simulink model "martins_version_wconv_wdc_wWT"  (R2023b)
settings: Solver=VariableStepAuto  StartTime=0.0  StopTime=30  RelTol=1.0e-3
undefined symbols (not defined in the file): C_dc, c_drt, c_f, C_hv_km, C_p_opt, Cagg, DiscIntNeverNeededParam, G_dc_denom, G_dc_num, H_gen, H_vsm, H_WTR, Ibase_hv, Ibase_lv, Ibase_mv, k_AD, k_d_vsm, k_decouple, k_drt, k_ffv, k_ic, k_idc, k_mod, k_p_p_vsm, k_p_q_vsm, k_pc, k_pdc, K_pitch, ki_dc, KI_LL, ki_q, kp_dc, KP_LL, kslope_VSC, L_comp, L_d, l_f, l_f_si1, l_grid, L_hv_km, L_q, l_t_ehvhv, l_t_hvmv, l_t_mvlv, L_Virt, Lagg, lambda_opt, Lbase1v, length_export, omega_nom, omega_WTR_min, omega_WTR_n, omega_WTR_sl, P_aero_0, phase_shift_test_state, phase_shifts, pie_export, pitch_max, pitch_min, Pitchanglevector ... (+40)
libraries: slpidlib x9, spsFirstOrderFilterLib x3, simulink x1, spsSampleandHoldLib x1, spspowerguiLib x1
(part 2 of 4)

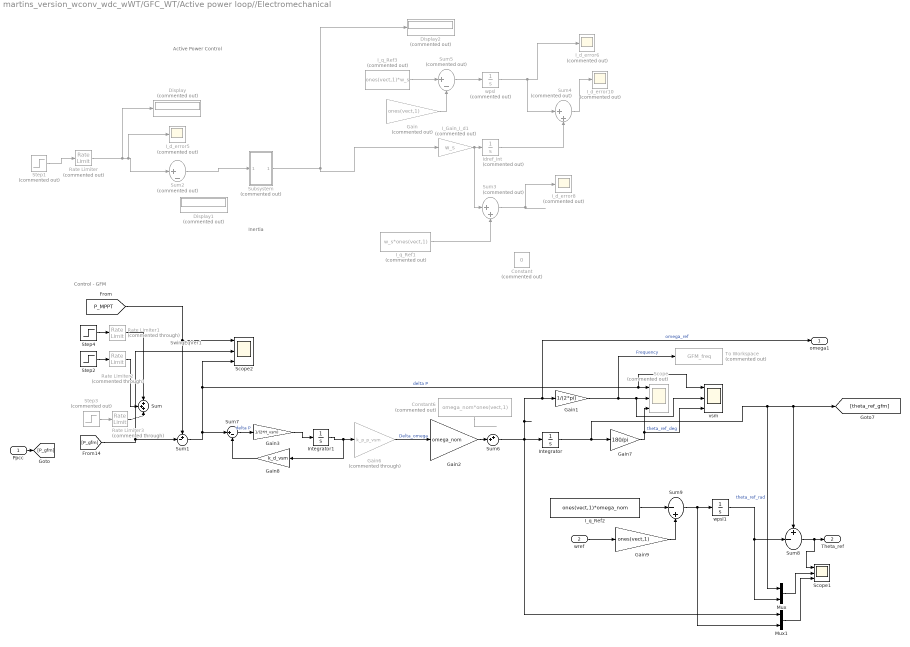
== system martins_version_wconv_wdc_wWT/GFC_WT/Active power loop//Electromechanical ==
  note: SwingEqVer1
  note: Active Power Control
  note: Inertia
  note: Control - GFM
  Ppcc : Inport  PortDimensions=vect
  wref : Inport  Port=2
  Constant : Constant  Commented=on  Value=0
  Constant6 : Constant  Commented=on  Value=omega_nom*ones(vect,1)
  Display : Display  Commented=on
  Display1 : Display  Commented=on
  Display2 : Display  Commented=on
  Gain : Gain  Commented=on  Gain=ones(vect,1)
  Gain1 : Gain  Gain=1/(2*pi)
  Gain2 : Gain  Gain=omega_nom
  Gain3 : Gain  Gain=1/(2*H_vsm)
  Gain6 : Gain  Commented=through  Gain=k_p_p_vsm
  Gain7 : Gain  Gain=180/pi
  Gain8 : Gain  Gain=k_d_vsm
  Gain9 : Gain  Gain=ones(vect,1)
  I_Gain_I_d1 : Gain  Commented=on  Gain=w_s
  I_d_error{5..6,8,10} (4 alike) : Scope  Commented=on
  I_q_Ref1 : Constant  Commented=on  Value=w_s*ones(vect,1)  SampleTime=-1
  I_q_Ref2 : Constant  Value=ones(vect,1)*omega_nom  SampleTime=-1
  I_q_Ref3 : Constant  Commented=on  Value=ones(vect,1)*w_s  SampleTime=-1
  "Idref_int " : Integrator  Commented=on  UpperSaturationLimit=300  LowerSaturationLimit=-100
  Integrator : Integrator  WrappedStateUpperValue=2*pi  WrappedStateLowerValue=0
  Integrator1 : Integrator
  Mux : Mux  Inputs=2
  Mux1 : Mux  Inputs=2
  Rate Limiter : RateLimiter  Commented=on  RisingSlewLimit=0.5  FallingSlewLimit=-0.5  SampleTimeMode=inherited
  Rate Limiter1 : RateLimiter  Commented=through  RisingSlewLimit=0.2  FallingSlewLimit=-0.2  SampleTimeMode=inherited
  Rate Limiter2 : RateLimiter  Commented=through  RisingSlewLimit=0.2  FallingSlewLimit=-0.2  SampleTimeMode=inherited
  Rate Limiter3 : RateLimiter  Commented=through  RisingSlewLimit=0.2  FallingSlewLimit=-0.2  SampleTimeMode=inherited
  Scope : Scope  Commented=on  NumInputPorts=3
  Scope1 : Scope  NumInputPorts=3
  Scope2 : Scope  NumInputPorts=3
  Step1 : Step  Commented=on  Time=2  Before=ones(vect,1)*0  After=ones(vect,1)*0.9  SampleTime=0
  Step2 : Step  Time=Tchange_gfm_ref+5  Before=0.0*ones(vect,1)  After=P_aero_0/2*ones(vect,1)  SampleTime=0
  Step3 : Step  Commented=on  Time=41  Before=0.0*ones(vect,1)  After=0.1*ones(vect,1)  SampleTime=0
  Step4 : Step  Time=Tchange_gfm_ref-1  Before=0.0*ones(vect,1)  After=P_aero_0/2*ones(vect,1)  SampleTime=0
  Subsystem : Subsystem  Commented=on
  Sum : Sum  Inputs=+++
  Sum1 : Sum  Inputs=+-|
  Sum2 : Sum  Commented=on  Inputs=|+-
  Sum3 : Sum  Commented=on  Inputs=|++
  Sum4 : Sum  Commented=on  Inputs=|++
  Sum5 : Sum  Commented=on  Inputs=|+-
  Sum6 : Sum  Inputs=++|
  Sum7 : Sum  Inputs=|+-
  Sum8 : Sum  Inputs=+-|
  Sum9 : Sum  Inputs=|-+
  To Workspace : ToWorkspace  Commented=on  VariableName=GFM_freq  SaveFormat=Structure With Time  SampleTime=-1
  vsm : Scope  NumInputPorts=3
  wpsl : Integrator  Commented=on  UpperSaturationLimit=300  LowerSaturationLimit=-100
  wpsl1 : Integrator  UpperSaturationLimit=300  LowerSaturationLimit=-100
  omega1 : Outport
  Theta_ref : Outport  Port=2
  wires:
  Subsystem/1(Out1) -> I_Gain_I_d1/1, Display2/1
  Sum4/1 -> I_d_error10/1
  I_Gain_I_d1/1 -> "Idref_int "/1, Sum3/1
  I_q_Ref3/1 -> Sum5/1
  ? -> Gain/1
  Sum5/1 -> wpsl/1
  wpsl/1 -> I_d_error6/1, Sum4/1
  I_q_Ref1/1 -> Sum3/2
  Sum3/1 -> I_d_error8/1
  "Idref_int "/1 -> Sum4/2
  Rate Limiter/1 -> I_d_error5/1, Sum2/1, Display/1
  Sum2/1 -> Subsystem/1(In1)
  Step1/1 -> Rate Limiter/1
  Gain/1 -> Sum5/2
  Step4/1 -> Rate Limiter1/1
  Ppcc/1 -> [P_gfm]
  Gain1/1 -> To Workspace/1, vsm/2, Scope/2  "Frequency"
  Gain2/1 -> Sum6/2
  Constant6/1 -> ?
  [P_MPPT] -> Sum1/1, Scope2/1
  Gain7/1 -> vsm/3, Scope/3  "theta_ref_deg"
  Gain6/1 -> Gain2/1  "Delta_omega"
  Sum6/1 -> Mux1/1, omega1/1, Gain1/1, Integrator/1  "omega_ref"
  Integrator/1 -> Mux/1, Sum8/1, [theta_ref_gfm], Gain7/1  "theta_ref_rad"
  Sum1/1 -> vsm/1, Scope/1, Scope2/3, Sum7/1  "delta P"
  Gain3/1 -> Integrator1/1
  Sum7/1 -> Gain3/1  "delta P"
  Gain8/1 -> Sum7/2
  Integrator1/1 -> Gain6/1, Gain8/1
  wref/1 -> Gain9/1
  wpsl1/1 -> Mux/2, Sum8/2
  I_q_Ref2/1 -> Sum9/1
  Gain9/1 -> Sum9/2
  Sum9/1 -> Mux1/2, wpsl1/1
  Sum8/1 -> Scope1/1, Theta_ref/1
  Mux/1 -> Scope1/2
  Mux1/1 -> Scope1/3
  [P_gfm] -> Sum1/2, Scope2/2
  Step2/1 -> Rate Limiter2/1
  Rate Limiter2/1 -> Sum/2
  Rate Limiter1/1 -> Sum/1
  Step3/1 -> Rate Limiter3/1
  Rate Limiter3/1 -> Sum/3

== system martins_version_wconv_wdc_wWT/GFC_WT/Current Limit Logic1 ==
  note: Circular Current limiter
  I_ref_unsat : Inport
  Abs1 : Abs
  Constant3 : Constant
  Constant4 : Constant  Value=1.2
  Demux6 : Demux  Outputs=2
  Demux7 : Demux  Outputs=[vect vect]
  Display3 : Display
  Divide : Product  Inputs=*/
  Divide1 : Product  Inputs=*/
  First-Order Filter1 : spsFirstOrderFilterLib/First-Order Filter  FilterType=Lowpass  Tc=0.002  Ts=0  Initialize=on  Vac_Init=[0, 0, 50]  Vdc_Init=0  PlotResponse=off  FreqRange="[0,  200,  1]"
  GreaterThan1 : RelationalOperator  Operator=>  OutDataTypeStr=boolean  RndMeth=Simplest  InputSameDT=off
  I_d_error2 : Scope  Commented=on
  I_d_error3 : Scope
  I_d_error5 : Scope  Commented=on
  Kip12 : Gain
  Kip13 : Gain  Gain=1/1.2
  Mux6 : Mux  Inputs=[vect vect]
  Real-Imag to Complex1 : RealImagToComplex
  Switch1 : Switch  Threshold=1  SaturateOnIntegerOverflow=off  InputSameDT=off
  Unit Delay2 : UnitDelay  InitialCondition=1  SampleTime=Ts_power  HasFrameUpgradeWarning=on
  Vmd2 : Display
  I_ref_sat : Outport
  wires:
  Mux6/1 -> I_ref_sat/1
  Divide1/1 -> Mux6/2
  Demux6/2 -> Real-Imag to Complex1/2
  Abs1/1 -> Kip13/1, I_d_error2/1, GreaterThan1/1
  Unit Delay2/1 -> Divide1/2, Divide/2
  Real-Imag to Complex1/1 -> Abs1/1
  Demux7/2 -> Divide1/1
  GreaterThan1/1 -> Switch1/2
  Demux6/1 -> Real-Imag to Complex1/1
  I_ref_unsat/1 -> Demux7/1, I_d_error5/1, Vmd2/1, First-Order Filter1/1
  Demux7/1 -> Divide/1
  Constant3/1 -> Switch1/3
  Kip13/1 -> Switch1/1
  Constant4/1 -> GreaterThan1/2
  Switch1/1 -> Kip12/1, I_d_error3/1
  Divide/1 -> Mux6/1
  Kip12/1 -> Display3/1, Unit Delay2/1
  First-Order Filter1/1 -> Demux6/1

== system martins_version_wconv_wdc_wWT/GFC_WT/CurrentControl ==
  ref : Inport
  meas : Inport  Port=2
  V grid meas : Inport  Port=3
  Constant : Constant
  Demux : Demux  Outputs=[vect vect]
  Demux1 : Demux  Outputs=[vect vect]
  Demux2 : Demux  Outputs=[vect vect]
  Divide1 : Product  Inputs=**
  Divide2 : Product  Inputs=**
  Gain4 : Gain  Gain=l_f
  Gain5 : Gain  Gain=l_f
  Mux : Mux  Inputs=[vect vect]
  Mux1 : Mux  Inputs=3
  Mux2 : Mux  Inputs=3
  PID Controller : slpidlib/PID Controller  Controller=PI  Form=Ideal  TimeDomain=Continuous-time  UseExternalTs=off  SampleTime=-1  IntegratorMethod=Forward Euler  FilterMethod=Forward Euler  ControllerParametersSource=internal  P=0.06  I=1/0.0013  UseKiTs=off  D=0  N=100  UseFilter=on  TunerSelectOption=Transfer Function Based (PID Tuner App)  InitialConditionSource=internal  InitialConditionForIntegrator=0  InitialConditionForFilter=0  DifferentiatorICPrevScaledInput=0  ExternalReset=none  TrackingMode=off  Kt=1  LimitOutput=off  SatLimitsSource=internal  UpperSaturationLimit=inf  LowerSaturationLimit=-inf  LinearizeAsGain=on  AntiWindupMode=none  Kb=1  LimitIntegrator=off  UpperIntegratorSaturationLimit=inf  LowerIntegratorSaturationLimit=-inf  POutMin=[]  POutMax=[]  IOutMin=[]  IOutMax=[]  DOutMin=[]  DOutMax=[]  NOutMin=[]  NOutMax=[]  SumOutMin=[]  SumOutMax=[]  SaturationOutMin=[]  SaturationOutMax=[]  PParamMin=[]  PParamMax=[]  IParamMin=[]  IParamMax=[]  DParamMin=[]  DParamMax=[]  NParamMin=[]  NParamMax=[]  KbParamMin=[]  KbParamMax=[]  KtParamMin=[]  KtParamMax=[]  KbOutMin=[]  KbOutMax=[]  KtOutMin=[]  KtOutMax=[]  IntegratorOutMin=[]  IntegratorOutMax=[]  FilterOutMin=[]  FilterOutMax=[]  SumI1OutMin=[]  SumI1OutMax=[]  SumI2OutMin=[]  SumI2OutMax=[]  SumI3OutMin=[]  SumI3OutMax=[]  SumI4OutMin=[]  SumI4OutMax=[]  SumDOutMin=[]  SumDOutMax=[]  DifferentiatorOutMin=[]  DifferentiatorOutMax=[]  FilterDiffOutCoefMin=[]  FilterDiffOutCoefMax=[]  ReciprocalOutMin=[]  ReciprocalOutMax=[]  SumDenOutMin=[]  SumDenOutMax=[]  SumNumOutMin=[]  SumNumOutMax=[]  DivideOutMin=[]  DivideOutMax=[]  UdiffTsProdOutMin=[]  UdiffTsProdOutMax=[]  NTsProdOutMin=[]  NTsProdOutMax=[]  UintegralTsProdOutMin=[]  UintegralTsProdOutMax=[]  UngainTsProdOutMin=[]  UngainTsProdOutMax=[]  ClampingZeroOutDataTypeStr=Inherit: Inherit via back propagation  ClampingZeroOutMin=[]  ClampingZeroOutMax=[]  FilterDenConstantOutDataTypeStr=Inherit: Inherit via back propagation  FilterDenConstantOutMin=[]  FilterDenConstantOutMax=[]  PCopyOutDataTypeStr=Inherit: Inherit via back propagation  PCopyOutMin=[]  PCopyOutMax=[]  NCopyOutDataTypeStr=Inherit: Inherit via back propagation  NCopyOutMin=[]  NCopyOutMax=[]  IntegratorContinuousStateAttributes=''  IntegratorStateMustResolveToSignalObject=off  IntegratorRTWStateStorageClass=Auto  FilterContinuousStateAttributes=''  FilterStateMustResolveToSignalObject=off  FilterRTWStateStorageClass=Auto  ParallelPVariant=Passthrough  IdealPVariant=InternalParameters  IVariant=InternalParameters  DVariant=Disabled  IntegratorVariant=Continuous  SatVariant=Disabled  AWVariant=Passthrough  PCopyVariant=Disabled  TRVariant=Disabled  FdbkBlocksVariant=Forward  IdealPFdbkVariant=Disabled  SatFdbkVariant=Disabled  DerivativeFilterVariant=Disabled  NVariant=Disabled  NCopyVariant=Disabled_SignalSpec  FilterICVariant=Disabled  IntegratorICVariant=InternalICs  ExternalResetVariant=Disabled  TRSumVariant=Passthrough  SumFdbkVariant=Disabled  SumVariant=Sum_PI  TsampFilterVariant=InternalTs  TsampNgainVariant=Passthrough  TsampIntegralVariant=Disabled_SignalSpec  ExternalSaturationOutDataTypeStr=Inherit: Same as second input
  PID Controller1 : slpidlib/PID Controller  Controller=PI  Form=Ideal  TimeDomain=Continuous-time  UseExternalTs=off  SampleTime=-1  IntegratorMethod=Forward Euler  FilterMethod=Forward Euler  ControllerParametersSource=internal  P=0.06  I=1/0.0013  UseKiTs=off  D=0  N=100  UseFilter=on  TunerSelectOption=Transfer Function Based (PID Tuner App)  InitialConditionSource=internal  InitialConditionForIntegrator=1  InitialConditionForFilter=0  DifferentiatorICPrevScaledInput=0  ExternalReset=none  TrackingMode=off  Kt=1  LimitOutput=off  SatLimitsSource=internal  UpperSaturationLimit=inf  LowerSaturationLimit=-inf  LinearizeAsGain=on  AntiWindupMode=none  Kb=1  LimitIntegrator=off  UpperIntegratorSaturationLimit=inf  LowerIntegratorSaturationLimit=-inf  POutMin=[]  POutMax=[]  IOutMin=[]  IOutMax=[]  DOutMin=[]  DOutMax=[]  NOutMin=[]  NOutMax=[]  SumOutMin=[]  SumOutMax=[]  SaturationOutMin=[]  SaturationOutMax=[]  PParamMin=[]  PParamMax=[]  IParamMin=[]  IParamMax=[]  DParamMin=[]  DParamMax=[]  NParamMin=[]  NParamMax=[]  KbParamMin=[]  KbParamMax=[]  KtParamMin=[]  KtParamMax=[]  KbOutMin=[]  KbOutMax=[]  KtOutMin=[]  KtOutMax=[]  IntegratorOutMin=[]  IntegratorOutMax=[]  FilterOutMin=[]  FilterOutMax=[]  SumI1OutMin=[]  SumI1OutMax=[]  SumI2OutMin=[]  SumI2OutMax=[]  SumI3OutMin=[]  SumI3OutMax=[]  SumI4OutMin=[]  SumI4OutMax=[]  SumDOutMin=[]  SumDOutMax=[]  DifferentiatorOutMin=[]  DifferentiatorOutMax=[]  FilterDiffOutCoefMin=[]  FilterDiffOutCoefMax=[]  ReciprocalOutMin=[]  ReciprocalOutMax=[]  SumDenOutMin=[]  SumDenOutMax=[]  SumNumOutMin=[]  SumNumOutMax=[]  DivideOutMin=[]  DivideOutMax=[]  UdiffTsProdOutMin=[]  UdiffTsProdOutMax=[]  NTsProdOutMin=[]  NTsProdOutMax=[]  UintegralTsProdOutMin=[]  UintegralTsProdOutMax=[]  UngainTsProdOutMin=[]  UngainTsProdOutMax=[]  ClampingZeroOutDataTypeStr=Inherit: Inherit via back propagation  ClampingZeroOutMin=[]  ClampingZeroOutMax=[]  FilterDenConstantOutDataTypeStr=Inherit: Inherit via back propagation  FilterDenConstantOutMin=[]  FilterDenConstantOutMax=[]  PCopyOutDataTypeStr=Inherit: Inherit via back propagation  PCopyOutMin=[]  PCopyOutMax=[]  NCopyOutDataTypeStr=Inherit: Inherit via back propagation  NCopyOutMin=[]  NCopyOutMax=[]  IntegratorContinuousStateAttributes=''  IntegratorStateMustResolveToSignalObject=off  IntegratorRTWStateStorageClass=Auto  FilterContinuousStateAttributes=''  FilterStateMustResolveToSignalObject=off  FilterRTWStateStorageClass=Auto  ParallelPVariant=Passthrough  IdealPVariant=InternalParameters  IVariant=InternalParameters  DVariant=Disabled  IntegratorVariant=Continuous  SatVariant=Disabled  AWVariant=Passthrough  PCopyVariant=Disabled  TRVariant=Disabled  FdbkBlocksVariant=Forward  IdealPFdbkVariant=Disabled  SatFdbkVariant=Disabled  DerivativeFilterVariant=Disabled  NVariant=Disabled  NCopyVariant=Disabled_SignalSpec  FilterICVariant=Disabled  IntegratorICVariant=InternalICs  ExternalResetVariant=Disabled  TRSumVariant=Passthrough  SumFdbkVariant=Disabled  SumVariant=Sum_PI  TsampFilterVariant=InternalTs  TsampNgainVariant=Passthrough  TsampIntegralVariant=Disabled_SignalSpec  ExternalSaturationOutDataTypeStr=Inherit: Same as second input
  Step1 : Step  Before=1  SampleTime=0
  Step2 : Step  Before=1  SampleTime=0
  Sum1 : Sum  Inputs=|+-
  Sum2 : Sum  Inputs=+-|
  Sum4 : Sum  Inputs=++-
  Sum5 : Sum  Inputs=+++
  Transfer Fcn2 : TransferFcn  Commented=on  Denominator=[0.005 1]
  Transfer Fcn3 : TransferFcn  Commented=on  Denominator=[0.005 1]
  d-axis-control : Scope  NumInputPorts=3
  q-axis control : Scope  NumInputPorts=3
  Out1 : Outport
  wires:
  Step2/1 -> Divide1/2
  Sum2/1 -> q-axis control/1, Divide1/1
  Mux2/1 -> q-axis control/2
  PID Controller1/1 -> Sum4/2, Mux1/2
  Step1/1 -> Divide2/2
  Divide2/1 -> PID Controller1/1
  Divide1/1 -> PID Controller/1
  Transfer Fcn3/1 -> Mux2/1, Sum5/3
  ref/1 -> Demux/1
  Gain4/1 -> Mux2/3, Sum5/1
  Transfer Fcn2/1 -> Mux1/1, Sum4/1
  Gain5/1 -> Mux1/3, Sum4/3
  V grid meas/1 -> Demux2/1
  Mux1/1 -> d-axis-control/2
  Sum4/1 -> d-axis-control/3, Mux/1
  Demux2/2 -> Transfer Fcn3/1
  Sum5/1 -> q-axis control/3, Mux/2
  PID Controller/1 -> Mux2/2, Sum5/2
  meas/1 -> Demux1/1
  Demux/1 -> Sum1/1
  Mux/1 -> Out1/1
  Demux/2 -> Sum2/1
  Demux1/1 -> Gain4/1, Sum1/2
  Demux1/2 -> Gain5/1, Sum2/2
  Sum1/1 -> Divide2/1, d-axis-control/1
  Demux2/1 -> Transfer Fcn2/1

== system martins_version_wconv_wdc_wWT/GFC_WT/DC-link voltage controller ==
  ref : Inport
  meas : Inport  Port=2
  G_dc : TransferFcn  Commented=on  Numerator=G_dc_num{1}  Denominator=G_dc_denom{1}
  Gain : Gain
  Gain1 : Gain
  Gain2 : Gain  Gain=-1
  Hit Crossing : HitCross
  Mux : Mux  Inputs=2
  PID Controller : slpidlib/PID Controller  Controller=PI  Form=Parallel  TimeDomain=Continuous-time  UseExternalTs=off  SampleTime=-1  IntegratorMethod=Forward Euler  FilterMethod=Forward Euler  ControllerParametersSource=internal  P=20  I=5  UseKiTs=off  D=0  N=100  UseFilter=on  TunerSelectOption=Transfer Function Based (PID Tuner App)  InitialConditionSource=internal  InitialConditionForIntegrator=0  InitialConditionForFilter=0  DifferentiatorICPrevScaledInput=0  ExternalReset=none  TrackingMode=off  Kt=1  LimitOutput=off  SatLimitsSource=internal  UpperSaturationLimit=0.5  LowerSaturationLimit=-0.5  LinearizeAsGain=on  AntiWindupMode=clamping  Kb=1  LimitIntegrator=off  UpperIntegratorSaturationLimit=0.5  LowerIntegratorSaturationLimit=-0.5  POutMin=[]  POutMax=[]  IOutMin=[]  IOutMax=[]  DOutMin=[]  DOutMax=[]  NOutMin=[]  NOutMax=[]  SumOutMin=[]  SumOutMax=[]  SaturationOutMin=[]  SaturationOutMax=[]  PParamMin=[]  PParamMax=[]  IParamMin=[]  IParamMax=[]  DParamMin=[]  DParamMax=[]  NParamMin=[]  NParamMax=[]  KbParamMin=[]  KbParamMax=[]  KtParamMin=[]  KtParamMax=[]  KbOutMin=[]  KbOutMax=[]  KtOutMin=[]  KtOutMax=[]  IntegratorOutMin=[]  IntegratorOutMax=[]  FilterOutMin=[]  FilterOutMax=[]  SumI1OutMin=[]  SumI1OutMax=[]  SumI2OutMin=[]  SumI2OutMax=[]  SumI3OutMin=[]  SumI3OutMax=[]  SumI4OutMin=[]  SumI4OutMax=[]  SumDOutMin=[]  SumDOutMax=[]  DifferentiatorOutMin=[]  DifferentiatorOutMax=[]  FilterDiffOutCoefMin=[]  FilterDiffOutCoefMax=[]  ReciprocalOutMin=[]  ReciprocalOutMax=[]  SumDenOutMin=[]  SumDenOutMax=[]  SumNumOutMin=[]  SumNumOutMax=[]  DivideOutMin=[]  DivideOutMax=[]  UdiffTsProdOutMin=[]  UdiffTsProdOutMax=[]  NTsProdOutMin=[]  NTsProdOutMax=[]  UintegralTsProdOutMin=[]  UintegralTsProdOutMax=[]  UngainTsProdOutMin=[]  UngainTsProdOutMax=[]  ClampingZeroOutDataTypeStr=Inherit: Inherit via back propagation  ClampingZeroOutMin=[]  ClampingZeroOutMax=[]  FilterDenConstantOutDataTypeStr=Inherit: Inherit via back propagation  FilterDenConstantOutMin=[]  FilterDenConstantOutMax=[]  PCopyOutDataTypeStr=Inherit: Inherit via back propagation  PCopyOutMin=[]  PCopyOutMax=[]  NCopyOutDataTypeStr=Inherit: Inherit via back propagation  NCopyOutMin=[]  NCopyOutMax=[]  IntegratorContinuousStateAttributes='dc_controller_man'  IntegratorStateMustResolveToSignalObject=off  IntegratorRTWStateStorageClass=Auto  FilterContinuousStateAttributes=''  FilterStateMustResolveToSignalObject=off  FilterRTWStateStorageClass=Auto  ParallelPVariant=InternalParameters  IdealPVariant=Disabled  IVariant=InternalParameters  DVariant=Disabled  IntegratorVariant=Continuous  SatVariant=Disabled  AWVariant=Passthrough  PCopyVariant=Disabled  TRVariant=Disabled  FdbkBlocksVariant=Forward  IdealPFdbkVariant=Disabled  SatFdbkVariant=Disabled  DerivativeFilterVariant=Disabled  NVariant=Disabled  NCopyVariant=Disabled_SignalSpec  FilterICVariant=Disabled  IntegratorICVariant=InternalICs  ExternalResetVariant=Disabled  TRSumVariant=Passthrough  SumFdbkVariant=Disabled  SumVariant=Sum_PI  TsampFilterVariant=InternalTs  TsampNgainVariant=Passthrough  TsampIntegralVariant=Disabled_SignalSpec  ExternalSaturationOutDataTypeStr=Inherit: Same as second input
  Square : Math  Operator=square
  Square1 : Math  Operator=square
  Square2 : Math  Commented=through  Operator=square
  Step : Step  Time=1.5  Before=1  After=0  SampleTime=0
  Sum : Sum  Inputs=+-|
  Switch : Switch  Criteria=u2 > Threshold  SaturateOnIntegerOverflow=off  InputSameDT=off
  v_dc_reg : Subsystem
  input : Outport
  error : Outport  Port=2
  out : Outport  Port=3
  DC_control : Outport  Port=4
  wires:
  Mux/1 -> Square2/1
  Gain/1 -> DC_control/1
  Sum/1 -> G_dc/1, v_dc_reg/1(In1), Gain1/1, Hit Crossing/1, error/1
  meas/1 -> Square/1
  ref/1 -> Square1/1
  Square/1 -> Mux/2, Sum/2
  Square1/1 -> Mux/1, Sum/1
  Hit Crossing/1 -> ?
  v_dc_reg/1(W) -> out/1, Gain/1, Switch/1
  Gain1/1 -> PID Controller/1
  Step/1 -> Switch/2
  G_dc/1 -> Gain2/1
  Gain2/1 -> Switch/3
  Square2/1 -> input/1

== system martins_version_wconv_wdc_wWT/GFC_WT/PLL>>grid1 ==
  note: inv ([  cos(wt)   sin(wt)
      |    -sin(wt)    cos(wt)   ])
  note: =
  note: [  al
      |     be  ]
  note: =
  note: [  al
      |     be  ]
  note: [ d
      |    q ]
  note: *
  note: [ d
      |    q ]
  note: [  cos(wt)   -sin(wt)
      |    sin(wt)    cos(wt)   ]
  note: *
  vgdq : Inport
  thetaPLL : Inport  Port=2
  Cos : Trigonometry  Operator=cos
  Demux1 : Demux  Outputs=2
  Display5 : Display
  Mux3 : Mux  Inputs=2
  Product{,1..3} (4 alike) : Product
  Sin : Trigonometry
  Sum : Sum  Inputs=+-
  Sum1 : Sum
  vgDQ : Outport  InitialOutput=[0,0]  VectorParamsAs1DForOutWhenUnconnected=off
  wires:
  vgdq/1 -> Demux1/1
  thetaPLL/1 -> Cos/1, Sin/1
  Sin/1 -> Product3/2, Product1/2
  Demux1/1 -> Product3/1, Product/1
  Cos/1 -> Product2/2, Product/2
  Product/1 -> Sum/1
  Demux1/2 -> Product2/1, Product1/1
  Product1/1 -> Sum/2
  Sum/1 -> Mux3/1
  Product2/1 -> Sum1/1
  Product3/1 -> Sum1/2
  Sum1/1 -> Mux3/2
  Mux3/1 -> Display5/1, vgDQ/1

== system martins_version_wconv_wdc_wWT/GFC_WT/PQ PCC ==
  note: PQ VSC bus
  IDQ : Inport
  VDQ : Inport  Port=2
  Demux7 : Demux  Outputs=[vect vect]
  Demux8 : Demux  Outputs=[vect vect]
  Product{1,3..5} (4 alike) : Product  InputSameDT=on  SaturateOnIntegerOverflow=on  OutDataTypeStr=Inherit: Same as first input
  Sum : Sum  InputSameDT=on  SaturateOnIntegerOverflow=on  OutDataTypeStr=Inherit: Same as first input
  Sum1 : Sum  Inputs=+-  InputSameDT=on  SaturateOnIntegerOverflow=on  OutDataTypeStr=Inherit: Same as first input
  P : Outport
  Q : Outport  Port=2
  wires:
  Product5/1 -> Sum1/2
  Product1/1 -> Sum1/1
  Demux8/2 -> Product1/1, Product4/1
  Demux7/1 -> Product1/2, Product3/1
  Demux8/1 -> Product5/1, Product3/2
  Product4/1 -> Sum/2
  Demux7/2 -> Product4/2, Product5/2
  Product3/1 -> Sum/1
  VDQ/1 -> Demux8/1
  Sum1/1 -> Q/1
  IDQ/1 -> Demux7/1
  Sum/1 -> P/1

== system martins_version_wconv_wdc_wWT/GFC_WT/PQ PCC1 ==
  note: PQ VSC bus
  IDQ : Inport
  VDQ : Inport  Port=2
  Demux7 : Demux  Outputs=[vect vect]
  Demux8 : Demux  Outputs=[vect vect]
  Product{1,3..5} (4 alike) : Product  InputSameDT=on  SaturateOnIntegerOverflow=on  OutDataTypeStr=Inherit: Same as first input
  Sum : Sum  InputSameDT=on  SaturateOnIntegerOverflow=on  OutDataTypeStr=Inherit: Same as first input
  Sum1 : Sum  Inputs=+-  InputSameDT=on  SaturateOnIntegerOverflow=on  OutDataTypeStr=Inherit: Same as first input
  P : Outport
  Q : Outport  Port=2
  wires:
  Product5/1 -> Sum1/2
  Product1/1 -> Sum1/1
  Demux8/2 -> Product1/1, Product4/1
  Demux7/1 -> Product1/2, Product3/1
  Demux8/1 -> Product5/1, Product3/2
  Product4/1 -> Sum/2
  Demux7/2 -> Product4/2, Product5/2
  Product3/1 -> Sum/1
  VDQ/1 -> Demux8/1
  Sum1/1 -> Q/1
  IDQ/1 -> Demux7/1
  Sum/1 -> P/1

== system martins_version_wconv_wdc_wWT/GFC_WT/PQ Virtual Bus1 ==
  note: PQ Virtual bus
  IDQ : Inport
  VDQ : Inport  Port=2
  Demux5 : Demux  Outputs=[vect vect]
  Demux6 : Demux  Outputs=[vect vect]
  Product{1,3..5} (4 alike) : Product  InputSameDT=on  SaturateOnIntegerOverflow=on  OutDataTypeStr=Inherit: Same as first input
  Sum : Sum  InputSameDT=on  SaturateOnIntegerOverflow=on  OutDataTypeStr=Inherit: Same as first input
  Sum1 : Sum  Inputs=+-  InputSameDT=on  SaturateOnIntegerOverflow=on  OutDataTypeStr=Inherit: Same as first input
  P : Outport
  Q : Outport  Port=2
  wires:
  Sum/1 -> P/1
  VDQ/1 -> Demux6/1
  IDQ/1 -> Demux5/1
  Sum1/1 -> Q/1
  Product5/1 -> Sum1/2
  Product1/1 -> Sum1/1
  Demux6/2 -> Product4/1, Product1/1
  Demux5/1 -> Product1/2, Product3/1
  Demux6/1 -> Product3/2, Product5/1
  Product4/1 -> Sum/2
  Demux5/2 -> Product5/2, Product4/2
  Product3/1 -> Sum/1

== system martins_version_wconv_wdc_wWT/GFC_WT/RL filter1 ==
  note: Inverter side inductor
  In1 : Inport
  In2 : Inport  Port=2
  In3 : Inport  Port=3
  In4 : Inport  Port=4
  In5 : Inport  Port=5
  1 : Gain  Gain=r_f*Zbase1v
  2 : Gain  Gain=1/(l_f*Lbase1v)
  3 : Gain  Gain=r_f*Zbase1v
  4 : Gain  Gain=1/(l_f*Lbase1v)
  Id : Scope
  Id_int : Integrator  UpperSaturationLimit=50  LowerSaturationLimit=-1000
  Iq : Scope
  Iq_int : Integrator  UpperSaturationLimit=50  LowerSaturationLimit=-1000
  L value : Constant  Value=l_f*Lbase1v  SampleTime=-1
  Product : Product
  Product1 : Product
  Product2 : Product
  Sum1 : Sum  Inputs=|+---
  Sum8 : Sum  Inputs=|+-+-
  id1 : Display
  Out1 : Outport
  Out2 : Outport  Port=2
  wires:
  In5/1 -> Product/1
  Product/1 -> [wL], id1/1
  L value/1 -> Product/2
  In1/1 -> Sum1/2
  In3/1 -> Sum1/1
  In4/1 -> Sum8/2
  In2/1 -> Sum8/1
  Product2/1 -> Sum8/3
  Iq_int/1 -> 3/1, Iq/1, Product2/2, Out1/1
  4/1 -> Iq_int/1
  Sum8/1 -> 2/1
  2/1 -> Id_int/1
  Sum1/1 -> 4/1
  3/1 -> Sum1/4
  Product1/1 -> Sum1/3
  1/1 -> Sum8/4
  Id_int/1 -> Product1/2, Out2/1, Id/1, 1/1
  [wL] -> Product1/1, Product2/1

== system martins_version_wconv_wdc_wWT/GFC_WT/Reactive Power //AVR ==
  note: Voltage control
  note: IQref
  Vmag : Inport
  Qmeas : Inport  Port=2
  Constant5 : Constant
  Gain1 : Gain
  Gain3 : Gain  Gain=ki_q
  Gain8 : Gain  Commented=through  Gain=1/Sbase1
  Gain9 : Gain  Gain=k_p_q_vsm
  I_Gain_I_d3 : Gain  Commented=on  Gain=kslope_VSC
  I_d_error{1,3..5} (4 alike) : Scope  Commented=on
  I_q_Ref1 : Constant  Commented=on  Value=ones(vect,1)  SampleTime=-1
  Integrator : Integrator  Commented=on  LimitOutput=on  UpperSaturationLimit=0.2  LowerSaturationLimit=-0.2
  Integrator1 : Integrator
  Kip1 : Gain  Commented=on  Gain=10
  Qdroop : Scope  NumInputPorts=2
  Qmeas1 : InportShadow  Port=2
  Qref1 : Constant  Value=0.0
  Scope : Scope  NumInputPorts=4
  Scope7 : Scope  Commented=on  NumInputPorts=2
  Step : Step  Commented=on  Time=2  Before=1  SampleTime=0
  Step2 : Step  Commented=on  Time=2  After=0  SampleTime=0
  Sum1 : Sum  Commented=on  Inputs=|+-+
  Sum3 : Sum  Inputs=|-+
  Sum4 : Sum  Inputs=|++
  Sum7 : Sum  Inputs=|+-
  Transfer Fcn1 : TransferFcn  Numerator=[ki_q]  Denominator=[1 ki_q]
  V_nominal : Constant  Value=ones(vect,1)
  Delta_V : Outport
  V_ref_d : Outport  Port=2
  wires:
  Kip1/1 -> Integrator/1
  Step/1 -> Sum1/1
  I_Gain_I_d3/1 -> Sum1/3, I_d_error5/1
  Qmeas/1 -> I_Gain_I_d3/1, I_d_error4/1
  Sum1/1 -> Kip1/1
  Integrator/1 -> I_d_error3/1, Delta_V/1
  Vmag/1 -> I_d_error1/1, Sum1/2
  [Q_grid] -> Gain8/1  "Gen Reactive Power"
  Qmeas1/1 -> [Q_grid]
  V_nominal/1 -> Sum4/2
  Gain8/1 -> Sum3/1
  Qref1/1 -> Sum3/2
  Sum4/1 -> Scope7/1, Qdroop/1, V_ref_d/1, Scope/4  "Vref"
  Sum3/1 -> Sum7/1, Scope7/2, Qdroop/2, Scope/1  "delta Q"
  Gain9/1 -> Scope/3, Sum4/1
  Constant5/1 -> ?
  Gain3/1 -> Integrator1/1
  Sum7/1 -> Gain3/1
  Gain1/1 -> Sum7/2
  Integrator1/1 -> Scope/2, Gain9/1, Gain1/1

== system martins_version_wconv_wdc_wWT/GFC_WT/Subsystem ==
  In1 : Inport
  In2 : Inport  Port=2
  omega_PLL : Inport  Port=3
  omega_ref : Inport  Port=4
  In4 : Inport  Port=5
  Constant : Constant  Commented=on  Value=Tdelay*w_s
  Current Control : Subsystem  Commented=on
  Current Limit Logic : Subsystem  Commented=through
  Demux4 : Demux  Commented=on  Outputs=2
  First-Order Filter : spsFirstOrderFilterLib/First-Order Filter  Commented=on  FilterType=Lowpass  Tc=0.02  Ts=0  Initialize=on  Vac_Init=[0, 0, 60]  Vdc_Init=0  PlotResponse=off  FreqRange="[0,  200,  1]"
  From1 : From  Commented=on  GotoTag=Idq
  From17 : From  Commented=on  GotoTag=vQ
  From18 : From  Commented=on  GotoTag=vD
  From2 : From  Commented=on  GotoTag=thetaPLL
  From4 : From  Commented=on  GotoTag=vdq
  From5 : From  Commented=on  GotoTag=Iodq
  Goto3 : Goto  Commented=on  GotoTag=IQ
  Goto4 : Goto  Commented=on  GotoTag=ID
  I_d_error4 : Scope  Commented=on
  Kip6 : Gain  Commented=on  Gain=Vbase_lv
  Kip9 : Gain  Commented=through  Gain=1/Vbase_lv_pk
  PLL>>grid2 : Subsystem  Commented=on  AncestorBlock=powerlib_meascontrol/Transformations/Alpha-Beta-Zero to dq0/Subsystem - pi//2 delay
  Product : Product  Commented=on  Inputs=**  InputSameDT=on  SaturateOnIntegerOverflow=on  OutDataTypeStr=Inherit: Same as first input
  RL filter : Subsystem  Commented=on
      settings: PortSchema="{\"entries\":[{\"content\":{\"sides\":[{\"content\":{\"connectorIds\":[\"In1\",\"In2\",\"In3\",\"In4\"]},\"type\":\"ConnectorPlacement.EquallySpacedRectSide\",\"uuid\":\"57ad71d1-5664-4b35-a20c-d71f7e1cdc47\"},{\"content\":{\"connectorIds\":[\"Out1\",\"Out2\"],\"side\":\"RIGHT\"},\"type\":\"ConnectorPlacement.EquallySpacedRectSide\",\"uuid\":\"8101605d-eedb-4c26-847d-0cc0ce629d60\"},{\"content\":{\"connectorIds\":[],\"side\":\"TOP\"},\"type\":\"ConnectorPlacement.EquallySpacedRectSide\",\"uuid\":\"2627b00b-24a5-469a-be2d-9c3c8a1d2080\"},{\"content\":{\"connectorIds\":[\"In5\"],\"side\":\"BOTTOM\"},\"type\":\"ConnectorPlacement.EquallySpacedRectSide\",\"uuid\":\"fe553db7-7727-4a02-b1e7-5aedfb7840ee\"}]},\"type\":\"ConnectorPlacement.EquallySpacedConnector\",\"uuid\":\"f40200c8-ad5b-428c-8a4e-7641595b86c4\"}],\"packageUris\":[\"http://schema.mathworks.com/mf0/Connector/19700101\"],\"version\":\"1.0\"}"
  Step : Step  Commented=on  Before=1  After=0  SampleTime=0
  Sum1 : Sum  Commented=on  Inputs=|+-
  Sum2 : Sum  Commented=on  Inputs=|+-
  Switch : Switch  Commented=on  Criteria=u2 > Threshold  SaturateOnIntegerOverflow=off  InputSameDT=off
  Transport Delay : TransportDelay  Commented=on  DelayTime=Tdelay/2
  Transport Delay1 : TransportDelay  Commented=on  DelayTime=Tdelay/2
  Vdc value for converter AC output of 1 pu for m=1 : Constant  Commented=on  Value=1/k_mod
  Virtual Admittance1 : Subsystem  Commented=on
  Vmd13 : Display  Commented=on
  wires:
  Demux4/2 -> Transport Delay1/1
  Transport Delay/1 -> RL filter/2(In2)
  RL filter/2(Out2) -> Goto4/1
  Demux4/1 -> Transport Delay/1
  RL filter/1(Out1) -> Goto3/1
  Vdc value for converter AC output of 1 pu for m=1/1 -> Product/2
  Step/1 -> Switch/2
  Current Limit Logic/1(I_ref_sat) -> Current Control/1(i_cv_ref), Vmd13/1
  From17/1 -> RL filter/1(In1)
  omega_ref/1 -> RL filter/5(In5)
  From1/1 -> Current Control/3(i_o)
  Transport Delay1/1 -> RL filter/3(In3)
  Sum2/1 -> Virtual Admittance1/1(delvdq)
  Kip6/1 -> PLL>>grid2/1(vgdq)
  From4/1 -> Current Control/2(v_o)
  From18/1 -> RL filter/4(In4)
  Sum1/1 -> PLL>>grid2/2(thetaPLL)
  First-Order Filter/1 -> Current Limit Logic/1(I_ref_unsat)
  From2/1 -> Sum1/1
  Virtual Admittance1/1(Idqref) -> First-Order Filter/1
  Constant/1 -> Sum1/2
  From5/1 -> Current Control/4(i_cv)
  Switch/1 -> Product/1
  PLL>>grid2/1(vgDQ) -> I_d_error4/1, Demux4/1
  In1/1 -> Sum2/1, Switch/1
  Current Control/1(v_ref_dq) -> Switch/3
  Product/1 -> Kip6/1
  omega_PLL/1 -> Virtual Admittance1/2(omega_PLL)
  In2/1 -> Sum2/2
  Kip9/1 -> ?
  In4/1 -> Kip9/1

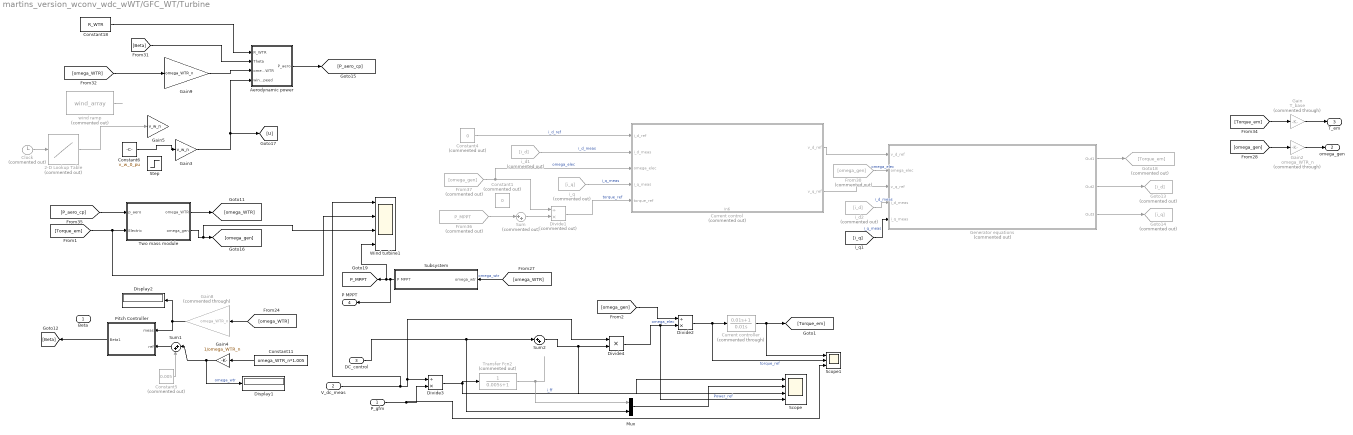
== system martins_version_wconv_wdc_wWT/GFC_WT/Turbine ==
  P_gfm : Inport
  V_dc_meas : Inport  Port=2
  DC_control : Inport  Port=3
  2-D Lookup Table : Lookup_n-D  Commented=on  NumberOfTableDimensions=1  BreakpointsForDimension1=wind_array_step(1,:)  BreakpointsForDimension2=[1:3]  IndexSearchMethod=Linear search  Table=wind_array_step(2,:)  InterpMethod=Nearest  InternalRulePriority=Speed  RndMeth=Simplest
  Aerodynamic power : Subsystem
  Clock : Clock  Commented=on
  Constant1 : Constant  Commented=on  Value=0
  Constant11 : Constant  Value=omega_WTR_n*1.005
  Constant18 : Constant  Value=R_WTR
  Constant4 : Constant  Commented=on  Value=0
  Constant5 : Constant  Commented=on  Value=0.005
  Constant6 : Constant  Value=v_w_0_pu
  Current control : Subsystem  Commented=on
      settings: PortSchema="{\"entries\":[{\"content\":{\"sides\":[{\"content\":{\"connectorIds\":[\"In1\",\"In2\",\"In3\",\"In4\",\"In5\"]},\"type\":\"ConnectorPlacement.EquallySpacedRectSide\",\"uuid\":\"f0c0ebaa-c967-4356-ac1b-c57f63a29779\"},{\"content\":{\"connectorIds\":[\"Out1\",\"Out2\"],\"side\":\"RIGHT\"},\"type\":\"ConnectorPlacement.EquallySpacedRectSide\",\"uuid\":\"1cdf54d9-8841-4054-96d8-98f023823611\"},{\"content\":{\"side\":\"TOP\"},\"type\":\"ConnectorPlacement.EquallySpacedRectSide\",\"uuid\":\"e5446ced-f102-4515-b1a2-d62d39d31328\"},{\"content\":{\"connectorIds\":[\"In6\"],\"side\":\"BOTTOM\"},\"type\":\"ConnectorPlacement.EquallySpacedRectSide\",\"uuid\":\"501a05db-372f-49fd-99c3-d79253c332da\"}]},\"type\":\"ConnectorPlacement.EquallySpacedConnector\",\"uuid\":\"99b5cc9b-ee78-4a5c-8cde-7a0c5c1e273f\"}],\"packageUris\":[\"http://schema.mathworks.com/mf0/Connector/R2020b\"],\"version\":\"1.0\"}"
  Current controller : TransferFcn  Commented=through  Numerator=[0.01 1]  Denominator=[0.01 0]
  Display1 : Display
  Display2 : Display
  Divide1 : Product  Commented=on  Inputs=/*
  Divide2 : Product  Inputs=/*
  Divide3 : Product  Inputs=/*
  Divide4 : Product  Inputs=**
  From30 : From  Commented=on  GotoTag=omega_gen
  From36 : From  Commented=on  GotoTag=P_MPPT
  From37 : From  Commented=on  GotoTag=omega_gen
  Gain : Gain  Commented=through  Gain=T_base
  Gain2 : Gain  Commented=through  Gain=omega_WTR_n
  Gain3 : Gain  Gain=v_w_n
  Gain4 : Gain  Gain=1/omega_WTR_n
  Gain5 : Gain  Gain=v_w_n
  Gain8 : Gain  Commented=through  Gain=omega_WTR_n
  Gain9 : Gain  Gain=omega_WTR_n
  Generator equations : Subsystem  Commented=on
  Goto13 : Goto  Commented=on  GotoTag=i_d
  Goto14 : Goto  Commented=on  GotoTag=i_q
  Goto18 : Goto  Commented=on  GotoTag=Torque_em
  Mux : Mux  Inputs=2
  Pitch Controller : Subsystem
  Scope : Scope  NumInputPorts=4
  Scope1 : Scope  NumInputPorts=3
  Step : Step  Time=4  Before=1  SampleTime=0
  Subsystem : Subsystem
  Sum : Sum  Commented=on  Inputs=|++
  Sum1 : Sum  Inputs=|++
  Sum2 : Sum  Inputs=|++
  Transfer Fcn2 : TransferFcn  Commented=on  Denominator=[0.005 1]
  Two mass module : Subsystem
  Wind turbine1 : Scope  NumInputPorts=4
  i_d1 : From  Commented=on  GotoTag=i_d
  i_d2 : From  Commented=on  GotoTag=i_d
  i_q : From  Commented=on  GotoTag=i_q
  wind ramp : FromWorkspace  Commented=on  VariableName=wind_array
  Beta : Outport
  omega_gen : Outport  Port=2
  T_em : Outport  Port=3
  P MPPT : Outport  Port=4
  tag scope: P_MPPT=global
  wires:
  [omega_gen] -> Gain2/1
  [omega_WTR] -> Subsystem/1(omega_wtr)  "omega_wtr"
  i_d1/1 -> Current control/2(i_d_meas)  "i_d_meas"
  Generator equations/3(Out3) -> Goto14/1
  [i_q] -> Generator equations/5(i_q_meas)  "i_q_meas"
  ? -> Beta/1
  i_d2/1 -> Generator equations/4(i_d_meas)  "i_d_meas"
  Constant18/1 -> Aerodynamic power/1(R_WTR)
  From30/1 -> Generator equations/2(omega_elec)  "omega_elec"
  Gain3/1 -> Aerodynamic power/4(wind speed), [U]
  [Torque_em] -> Wind turbine1/2, Two mass module/2(Electric)
  Constant11/1 -> Gain4/1
  wind ramp/1 -> ?
  [P_aero_cp] -> Two mass module/1(p_aero)
  Constant4/1 -> Current control/1(i_d_ref)  "i_d_ref"
  Generator equations/1(Out1) -> Goto18/1
  Constant5/1 -> Sum1/2
  Two mass module/1(omega_WTR) -> [omega_WTR]
  From36/1 -> Sum/1
  Two mass module/2(omega_gen) -> Wind turbine1/3, [omega_gen]
  From37/1 -> Divide1/1, Current control/3(omega_elec)  "omega_elec"
  Sum1/1 -> Pitch Controller/2(ref)
  Gain4/1 -> Sum1/1, Display1/1  "omega_wtr"
  Constant6/1 -> Gain3/1
  [omega_WTR] -> Gain8/1
  Clock/1 -> 2-D Lookup Table/1
  Pitch Controller/1(Beta1) -> [Beta]
  i_q/1 -> Current control/4(i_q_meas)  "i_q_meas"
  Aerodynamic power/1(P_aero) -> [P_aero_cp]
  Gain9/1 -> Aerodynamic power/3(omega_WTR)
  Gain8/1 -> Display2/1, Pitch Controller/1(meas)
  [Beta] -> Aerodynamic power/2(Theta)
  2-D Lookup Table/1 -> Gain5/1
  [Torque_em] -> Gain/1
  Subsystem/1(P MPPT) -> P MPPT/1, Wind turbine1/4, [P_MPPT]
  Divide1/1 -> Current control/5(torque_ref)  "torque_ref"
  Current control/1(v_d_ref) -> Generator equations/1(v_d_ref)
  Generator equations/2(Out2) -> Goto13/1
  [omega_WTR] -> Gain9/1
  Current control/2(v_q_ref) -> Generator equations/3(v_q_ref)
  Gain/1 -> T_em/1
  Gain2/1 -> omega_gen/1
  Sum/1 -> Divide1/2
  P_gfm/1 -> Scope1/3, Divide3/2
  DC_control/1 -> Sum2/1, Mux/2
  [omega_gen] -> Divide2/1  "omega_elec"
  Current controller/1 -> Scope1/1, [Torque_em]
  Divide2/1 -> Scope1/2, Current controller/1  "torque_ref"
  Divide3/1 -> Transfer Fcn2/1, Scope/1  "i_ff"
  Transfer Fcn2/1 -> Mux/1
  Sum2/1 -> Scope/3, Divide4/2
  Divide4/1 -> Scope/4, Divide2/2  "Power_ref"
  Mux/1 -> Scope/2
  V_dc_meas/1 -> Wind turbine1/1, Divide4/1, Divide3/1

== system martins_version_wconv_wdc_wWT/GFC_WT/VoltageControl ==
  ref : Inport
  meas : Inport  Port=2
  I filter meas : Inport  Port=3
  Constant : Constant  Value=0
  Demux1 : Demux  Outputs=[vect vect]
  Demux2 : Demux  Outputs=[vect vect]
  Demux3 : Demux  Outputs=[vect vect]
  Gain4 : Gain  Gain=c_f
  Gain5 : Gain  Gain=c_f
  Mux : Mux  Inputs=[vect vect]
  Mux1 : Mux  Inputs=3
  Mux2 : Mux  Inputs=3
  PID Controller : slpidlib/PID Controller  Controller=PI  Form=Parallel  TimeDomain=Continuous-time  UseExternalTs=off  SampleTime=-1  IntegratorMethod=Forward Euler  FilterMethod=Forward Euler  ControllerParametersSource=internal  P=0.479  I=1/0.007  UseKiTs=off  D=0  N=100  UseFilter=on  TunerSelectOption=Transfer Function Based (PID Tuner App)  InitialConditionSource=internal  InitialConditionForIntegrator=0  InitialConditionForFilter=0  DifferentiatorICPrevScaledInput=0  ExternalReset=none  TrackingMode=off  Kt=1  LimitOutput=off  SatLimitsSource=internal  UpperSaturationLimit=2  LowerSaturationLimit=-2  LinearizeAsGain=off  AntiWindupMode=none  Kb=1  LimitIntegrator=off  UpperIntegratorSaturationLimit=inf  LowerIntegratorSaturationLimit=-inf  POutMin=[]  POutMax=[]  IOutMin=[]  IOutMax=[]  DOutMin=[]  DOutMax=[]  NOutMin=[]  NOutMax=[]  SumOutMin=[]  SumOutMax=[]  SaturationOutMin=[]  SaturationOutMax=[]  PParamMin=[]  PParamMax=[]  IParamMin=[]  IParamMax=[]  DParamMin=[]  DParamMax=[]  NParamMin=[]  NParamMax=[]  KbParamMin=[]  KbParamMax=[]  KtParamMin=[]  KtParamMax=[]  KbOutMin=[]  KbOutMax=[]  KtOutMin=[]  KtOutMax=[]  IntegratorOutMin=[]  IntegratorOutMax=[]  FilterOutMin=[]  FilterOutMax=[]  SumI1OutMin=[]  SumI1OutMax=[]  SumI2OutMin=[]  SumI2OutMax=[]  SumI3OutMin=[]  SumI3OutMax=[]  SumI4OutMin=[]  SumI4OutMax=[]  SumDOutMin=[]  SumDOutMax=[]  DifferentiatorOutMin=[]  DifferentiatorOutMax=[]  FilterDiffOutCoefMin=[]  FilterDiffOutCoefMax=[]  ReciprocalOutMin=[]  ReciprocalOutMax=[]  SumDenOutMin=[]  SumDenOutMax=[]  SumNumOutMin=[]  SumNumOutMax=[]  DivideOutMin=[]  DivideOutMax=[]  UdiffTsProdOutMin=[]  UdiffTsProdOutMax=[]  NTsProdOutMin=[]  NTsProdOutMax=[]  UintegralTsProdOutMin=[]  UintegralTsProdOutMax=[]  UngainTsProdOutMin=[]  UngainTsProdOutMax=[]  ClampingZeroOutDataTypeStr=Inherit: Inherit via back propagation  ClampingZeroOutMin=[]  ClampingZeroOutMax=[]  FilterDenConstantOutDataTypeStr=Inherit: Inherit via back propagation  FilterDenConstantOutMin=[]  FilterDenConstantOutMax=[]  PCopyOutDataTypeStr=Inherit: Inherit via back propagation  PCopyOutMin=[]  PCopyOutMax=[]  NCopyOutDataTypeStr=Inherit: Inherit via back propagation  NCopyOutMin=[]  NCopyOutMax=[]  IntegratorContinuousStateAttributes=''  IntegratorStateMustResolveToSignalObject=off  IntegratorRTWStateStorageClass=Auto  FilterContinuousStateAttributes=''  FilterStateMustResolveToSignalObject=off  FilterRTWStateStorageClass=Auto  ParallelPVariant=InternalParameters  IdealPVariant=Disabled  IVariant=InternalParameters  DVariant=Disabled  IntegratorVariant=Continuous  SatVariant=Disabled  AWVariant=Passthrough  PCopyVariant=Disabled  TRVariant=Disabled  FdbkBlocksVariant=Forward  IdealPFdbkVariant=Disabled  SatFdbkVariant=Disabled  DerivativeFilterVariant=Disabled  NVariant=Disabled  NCopyVariant=Disabled_SignalSpec  FilterICVariant=Disabled  IntegratorICVariant=InternalICs  ExternalResetVariant=Disabled  TRSumVariant=Passthrough  SumFdbkVariant=Disabled  SumVariant=Sum_PI  TsampFilterVariant=InternalTs  TsampNgainVariant=Passthrough  TsampIntegralVariant=Disabled_SignalSpec  ExternalSaturationOutDataTypeStr=Inherit: Same as second input
  PID Controller1 : slpidlib/PID Controller  Controller=PI  Form=Ideal  TimeDomain=Continuous-time  UseExternalTs=off  SampleTime=-1  IntegratorMethod=Forward Euler  FilterMethod=Forward Euler  ControllerParametersSource=internal  P=0.479  I=1/0.007  UseKiTs=off  D=0  N=100  UseFilter=on  TunerSelectOption=Transfer Function Based (PID Tuner App)  InitialConditionSource=internal  InitialConditionForIntegrator=1  InitialConditionForFilter=0  DifferentiatorICPrevScaledInput=0  ExternalReset=none  TrackingMode=off  Kt=1  LimitOutput=off  SatLimitsSource=internal  UpperSaturationLimit=2  LowerSaturationLimit=-2  LinearizeAsGain=off  AntiWindupMode=none  Kb=1  LimitIntegrator=off  UpperIntegratorSaturationLimit=inf  LowerIntegratorSaturationLimit=-inf  POutMin=[]  POutMax=[]  IOutMin=[]  IOutMax=[]  DOutMin=[]  DOutMax=[]  NOutMin=[]  NOutMax=[]  SumOutMin=[]  SumOutMax=[]  SaturationOutMin=[]  SaturationOutMax=[]  PParamMin=[]  PParamMax=[]  IParamMin=[]  IParamMax=[]  DParamMin=[]  DParamMax=[]  NParamMin=[]  NParamMax=[]  KbParamMin=[]  KbParamMax=[]  KtParamMin=[]  KtParamMax=[]  KbOutMin=[]  KbOutMax=[]  KtOutMin=[]  KtOutMax=[]  IntegratorOutMin=[]  IntegratorOutMax=[]  FilterOutMin=[]  FilterOutMax=[]  SumI1OutMin=[]  SumI1OutMax=[]  SumI2OutMin=[]  SumI2OutMax=[]  SumI3OutMin=[]  SumI3OutMax=[]  SumI4OutMin=[]  SumI4OutMax=[]  SumDOutMin=[]  SumDOutMax=[]  DifferentiatorOutMin=[]  DifferentiatorOutMax=[]  FilterDiffOutCoefMin=[]  FilterDiffOutCoefMax=[]  ReciprocalOutMin=[]  ReciprocalOutMax=[]  SumDenOutMin=[]  SumDenOutMax=[]  SumNumOutMin=[]  SumNumOutMax=[]  DivideOutMin=[]  DivideOutMax=[]  UdiffTsProdOutMin=[]  UdiffTsProdOutMax=[]  NTsProdOutMin=[]  NTsProdOutMax=[]  UintegralTsProdOutMin=[]  UintegralTsProdOutMax=[]  UngainTsProdOutMin=[]  UngainTsProdOutMax=[]  ClampingZeroOutDataTypeStr=Inherit: Inherit via back propagation  ClampingZeroOutMin=[]  ClampingZeroOutMax=[]  FilterDenConstantOutDataTypeStr=Inherit: Inherit via back propagation  FilterDenConstantOutMin=[]  FilterDenConstantOutMax=[]  PCopyOutDataTypeStr=Inherit: Inherit via back propagation  PCopyOutMin=[]  PCopyOutMax=[]  NCopyOutDataTypeStr=Inherit: Inherit via back propagation  NCopyOutMin=[]  NCopyOutMax=[]  IntegratorContinuousStateAttributes=''  IntegratorStateMustResolveToSignalObject=off  IntegratorRTWStateStorageClass=Auto  FilterContinuousStateAttributes=''  FilterStateMustResolveToSignalObject=off  FilterRTWStateStorageClass=Auto  ParallelPVariant=Passthrough  IdealPVariant=InternalParameters  IVariant=InternalParameters  DVariant=Disabled  IntegratorVariant=Continuous  SatVariant=Disabled  AWVariant=Passthrough  PCopyVariant=Disabled  TRVariant=Disabled  FdbkBlocksVariant=Forward  IdealPFdbkVariant=Disabled  SatFdbkVariant=Disabled  DerivativeFilterVariant=Disabled  NVariant=Disabled  NCopyVariant=Disabled_SignalSpec  FilterICVariant=Disabled  IntegratorICVariant=InternalICs  ExternalResetVariant=Disabled  TRSumVariant=Passthrough  SumFdbkVariant=Disabled  SumVariant=Sum_PI  TsampFilterVariant=InternalTs  TsampNgainVariant=Passthrough  TsampIntegralVariant=Disabled_SignalSpec  ExternalSaturationOutDataTypeStr=Inherit: Same as second input
  Sum1 : Sum  Inputs=|+-
  Sum2 : Sum  Inputs=+-|
  Sum4 : Sum  Inputs=++-
  Sum5 : Sum  Inputs=+++
  Transfer Fcn2 : TransferFcn  Commented=on  Denominator=[0.005 1]
  Transfer Fcn3 : TransferFcn  Commented=on  Denominator=[0.005 1]
  d-axis v control : Scope  NumInputPorts=3
  q-axis v control : Scope  NumInputPorts=3
  I_ref_unsat : Outport
  wires:
  Mux2/1 -> d-axis v control/2
  Transfer Fcn2/1 -> Sum5/3, Mux1/1
  ? -> ?
  PID Controller1/1 -> Mux2/2, Sum4/2
  Mux1/1 -> q-axis v control/2
  Demux3/2 -> Sum2/1
  meas/1 -> Demux1/1
  Gain5/1 -> Mux1/3, Sum5/1
  PID Controller/1 -> Mux1/2, Sum5/2
  Demux2/2 -> Transfer Fcn2/1
  Sum5/1 -> Mux/2, q-axis v control/3
  Mux/1 -> I_ref_unsat/1
  Gain4/1 -> Mux2/3, Sum4/3
  Demux1/2 -> Gain4/1, Sum2/2
  Sum1/1 -> PID Controller1/1, d-axis v control/1
  Demux1/1 -> Sum1/2, Gain5/1
  ref/1 -> Demux3/1
  Sum2/1 -> PID Controller/1, q-axis v control/1
  Transfer Fcn3/1 -> Mux2/1, Sum4/1
  Demux2/1 -> Transfer Fcn3/1
  I filter meas/1 -> Demux2/1
  Sum4/1 -> Mux/1, d-axis v control/3
  Demux3/1 -> Sum1/1

== system martins_version_wconv_wdc_wWT/GFC_WT/grid>>PLL1 ==
  note: [  al
      |     be  ]
  note: [ d
      |    q ]
  note: [  cos(wt)   -sin(wt)
      |    sin(wt)    cos(wt)   ]
  note: =
  note: *
  note: [  al
      |     be  ]
  note: [ d
      |    q ]
  note: inv ([  cos(wt)   sin(wt)
      |    -sin(wt)    cos(wt)   ])
  note: =
  note: *
  vgDQ : Inport
  wt : Inport  Port=2
  Cos : Trigonometry  Operator=cos
  Demux1 : Demux  Outputs=[vect vect]
  Display5 : Display
  Mux3 : Mux  Inputs=2
  Product{,1..3} (4 alike) : Product
  Sin : Trigonometry
  Sum : Sum
  Sum1 : Sum  Inputs=+-
  vgdq : Outport  InitialOutput=[0,0]  VectorParamsAs1DForOutWhenUnconnected=off
  wires:
  Product3/1 -> Sum1/2
  Demux1/2 -> Product2/1, Product1/1
  Product2/1 -> Sum1/1
  Cos/1 -> Product2/2, Product/2
  Product1/1 -> Sum/2
  Sin/1 -> Product3/2, Product1/2
  vgDQ/1 -> Demux1/1
  Sum1/1 -> Mux3/2
  Mux3/1 -> vgdq/1, Display5/1
  Sum/1 -> Mux3/1
  Product/1 -> Sum/1
  wt/1 -> Cos/1, Sin/1
  Demux1/1 -> Product3/1, Product/1

== system martins_version_wconv_wdc_wWT/GFC_WT/grid>>PLL2 ==
  note: *
  note: =
  note: inv ([  cos(wt)   sin(wt)
      |    -sin(wt)    cos(wt)   ])
  note: [ d
      |    q ]
  note: [  al
      |     be  ]
  note: *
  note: =
  note: [  cos(wt)   -sin(wt)
      |    sin(wt)    cos(wt)   ]
  note: [ d
      |    q ]
  note: [  al
      |     be  ]
  vgDQ : Inport
  wt : Inport  Port=2
  Cos : Trigonometry  Operator=cos
  Demux1 : Demux  Outputs=2
  Display5 : Display
  Mux3 : Mux  Inputs=2
  Product{,1..3} (4 alike) : Product
  Sin : Trigonometry
  Sum : Sum
  Sum1 : Sum  Inputs=+-
  vgdq : Outport  InitialOutput=[0,0]  VectorParamsAs1DForOutWhenUnconnected=off
  wires:
  Demux1/1 -> Product/1, Product3/1
  wt/1 -> Sin/1, Cos/1
  Product/1 -> Sum/1
  Sum/1 -> Mux3/1
  Mux3/1 -> Display5/1, vgdq/1
  Sum1/1 -> Mux3/2
  vgDQ/1 -> Demux1/1
  Sin/1 -> Product1/2, Product3/2
  Product1/1 -> Sum/2
  Cos/1 -> Product/2, Product2/2
  Product2/1 -> Sum1/1
  Demux1/2 -> Product1/1, Product2/1
  Product3/1 -> Sum1/2

== system martins_version_wconv_wdc_wWT/GFC_WT/grid>>PLL3 ==
  note: *
  note: =
  note: inv ([  cos(wt)   sin(wt)
      |    -sin(wt)    cos(wt)   ])
  note: [ d
      |    q ]
  note: [  al
      |     be  ]
  note: *
  note: =
  note: [  cos(wt)   -sin(wt)
      |    sin(wt)    cos(wt)   ]
  note: [ d
      |    q ]
  note: [  al
      |     be  ]
  vgDQ : Inport
  wt : Inport  Port=2
  Cos : Trigonometry  Operator=cos
  Demux1 : Demux  Outputs=2
  Display5 : Display
  Mux3 : Mux  Inputs=[vect vect]
  Product{,1..3} (4 alike) : Product
  Sin : Trigonometry
  Sum : Sum
  Sum1 : Sum  Inputs=+-
  vgdq : Outport  InitialOutput=[0,0]  VectorParamsAs1DForOutWhenUnconnected=off
  wires:
  Demux1/1 -> Product/1, Product3/1
  wt/1 -> Sin/1, Cos/1
  Product/1 -> Sum/1
  Sum/1 -> Mux3/1
  Mux3/1 -> Display5/1, vgdq/1
  Sum1/1 -> Mux3/2
  vgDQ/1 -> Demux1/1
  Sin/1 -> Product1/2, Product3/2
  Product1/1 -> Sum/2
  Cos/1 -> Product/2, Product2/2
  Product2/1 -> Sum1/1
  Demux1/2 -> Product1/1, Product2/1
  Product3/1 -> Sum1/2

== system martins_version_wconv_wdc_wWT/GFC_WT/v_dc_reg ==
  In1 : Inport
  Ipart : DiscreteIntegrator  Commented=on  gainval=k_idc  SampleTime=-1  ICPrevOutput=DiscIntNeverNeededParam  ICPrevScaledInput=DiscIntNeverNeededParam
  PID Controller : slpidlib/PID Controller  Controller=PI  Form=Parallel  TimeDomain=Continuous-time  UseExternalTs=off  SampleTime=-1  IntegratorMethod=Forward Euler  FilterMethod=Forward Euler  ControllerParametersSource=internal  P=k_pdc  I=k_idc  UseKiTs=off  D=0  N=100  UseFilter=on  TunerSelectOption=Transfer Function Based (PID Tuner App)  InitialConditionSource=internal  InitialConditionForIntegrator=0  InitialConditionForFilter=0  DifferentiatorICPrevScaledInput=0  ExternalReset=none  TrackingMode=off  Kt=1  LimitOutput=off  SatLimitsSource=internal  UpperSaturationLimit=inf  LowerSaturationLimit=-inf  LinearizeAsGain=on  AntiWindupMode=none  Kb=1  LimitIntegrator=off  UpperIntegratorSaturationLimit=inf  LowerIntegratorSaturationLimit=-inf  POutMin=[]  POutMax=[]  IOutMin=[]  IOutMax=[]  DOutMin=[]  DOutMax=[]  NOutMin=[]  NOutMax=[]  SumOutMin=[]  SumOutMax=[]  SaturationOutMin=[]  SaturationOutMax=[]  PParamMin=[]  PParamMax=[]  IParamMin=[]  IParamMax=[]  DParamMin=[]  DParamMax=[]  NParamMin=[]  NParamMax=[]  KbParamMin=[]  KbParamMax=[]  KtParamMin=[]  KtParamMax=[]  KbOutMin=[]  KbOutMax=[]  KtOutMin=[]  KtOutMax=[]  IntegratorOutMin=[]  IntegratorOutMax=[]  FilterOutMin=[]  FilterOutMax=[]  SumI1OutMin=[]  SumI1OutMax=[]  SumI2OutMin=[]  SumI2OutMax=[]  SumI3OutMin=[]  SumI3OutMax=[]  SumI4OutMin=[]  SumI4OutMax=[]  SumDOutMin=[]  SumDOutMax=[]  DifferentiatorOutMin=[]  DifferentiatorOutMax=[]  FilterDiffOutCoefMin=[]  FilterDiffOutCoefMax=[]  ReciprocalOutMin=[]  ReciprocalOutMax=[]  SumDenOutMin=[]  SumDenOutMax=[]  SumNumOutMin=[]  SumNumOutMax=[]  DivideOutMin=[]  DivideOutMax=[]  UdiffTsProdOutMin=[]  UdiffTsProdOutMax=[]  NTsProdOutMin=[]  NTsProdOutMax=[]  UintegralTsProdOutMin=[]  UintegralTsProdOutMax=[]  UngainTsProdOutMin=[]  UngainTsProdOutMax=[]  ClampingZeroOutDataTypeStr=Inherit: Inherit via back propagation  ClampingZeroOutMin=[]  ClampingZeroOutMax=[]  FilterDenConstantOutDataTypeStr=Inherit: Inherit via back propagation  FilterDenConstantOutMin=[]  FilterDenConstantOutMax=[]  PCopyOutDataTypeStr=Inherit: Inherit via back propagation  PCopyOutMin=[]  PCopyOutMax=[]  NCopyOutDataTypeStr=Inherit: Inherit via back propagation  NCopyOutMin=[]  NCopyOutMax=[]  IntegratorContinuousStateAttributes=''  IntegratorStateMustResolveToSignalObject=off  IntegratorRTWStateStorageClass=Auto  FilterContinuousStateAttributes=''  FilterStateMustResolveToSignalObject=off  FilterRTWStateStorageClass=Auto  ParallelPVariant=InternalParameters  IdealPVariant=Disabled  IVariant=InternalParameters  DVariant=Disabled  IntegratorVariant=Continuous  SatVariant=Disabled  AWVariant=Passthrough  PCopyVariant=Disabled  TRVariant=Disabled  FdbkBlocksVariant=Forward  IdealPFdbkVariant=Disabled  SatFdbkVariant=Disabled  DerivativeFilterVariant=Disabled  NVariant=Disabled  NCopyVariant=Disabled_SignalSpec  FilterICVariant=Disabled  IntegratorICVariant=InternalICs  ExternalResetVariant=Disabled  TRSumVariant=Passthrough  SumFdbkVariant=Disabled  SumVariant=Sum_PI  TsampFilterVariant=InternalTs  TsampNgainVariant=Passthrough  TsampIntegralVariant=Disabled_SignalSpec  ExternalSaturationOutDataTypeStr=Inherit: Same as second input
  Ppart : Gain  Commented=on  Gain=k_pdc  SaturateOnIntegerOverflow=on  OutDataTypeStr=Inherit: Same as input  ParamDataTypeStr=Inherit: Same as input
  Sum5 : Sum  Commented=on  Inputs=|++  InputSameDT=on  SaturateOnIntegerOverflow=on  OutDataTypeStr=Inherit: Same as first input
  W : Outport
  wires:
  Ppart/1 -> Sum5/1
  Ipart/1 -> Sum5/2
  In1/1 -> PID Controller/1, Ppart/1, Ipart/1
  PID Controller/1 -> W/1
